simulink model "example_DHWconsumptionBasic"  (R2013b)
settings: Solver=ode45  StartTime=0.0  StopTime=24*3600  RelTol=1e-3
libraries: carnot x5
settings Model: Creator=drhf  LastModifiedBy=drhf
settings DataIOCC: SignalLoggingSaveFormat=ModelDataLogs
settings OptimizationCC: ExpressionDepthLimit=2147483647
settings DebuggingCC: FcnCallInpInsideContextMsg=UseLocalSettings  StateNameClashWarn=warning
settings GRTTargetCC: CombineOutputUpdateFcns=off  GRTInterface=on

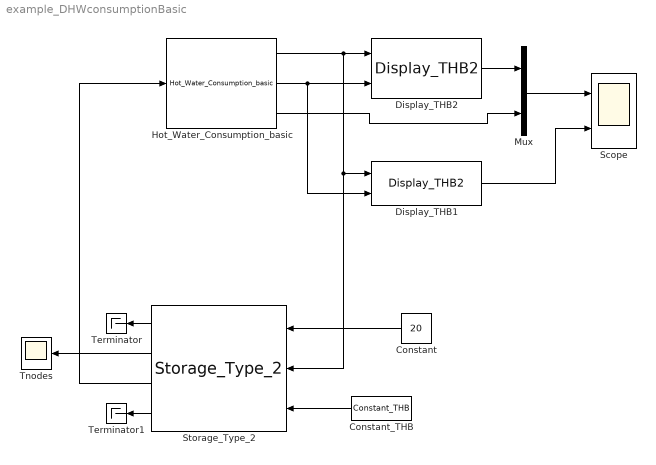
== system example_DHWconsumptionBasic ==
  Constant : Constant  Value=20
  Constant_THB : carnot/Source/Simple/Constant_THB  t=40  mdot=0*100/3600  p=1e5  mID=No Pressure Drop  fluid=Water  mix=0  mix2=0  mix3=0  dia=0.02  hgt=0
  Display_THB1 : carnot/Outputs/Display_THB2  t=off  m=on  p=off  id=off  mix=off  d=off
  Display_THB2 : carnot/Outputs/Display_THB2  t=on  m=off  p=off  id=off  mix=off  d=off
  Hot_Water_Consumption_basic : carnot/Load/Hot_Water_Tapping/Applications/Hot_Water_Consumption_basic  Thot=45  Tcold=10  period="24*3600   % one day"  time="[7 12 19]*3600  % tapping at 7:00, 12:00 and 19:00"  duration="[0.2 0.1 0.2]*3600  % in total 1/2 h tapping"  mdot="[1 1 1]*200/1800   % 200 kg in 1/2 h"
  Mux : Mux  Inputs=2
  Scope : Scope  NumInputPorts=2
      settings: YMin=5~0  YMax=55~0.12
  Storage_Type_2 : carnot/Storage/Thermal/Storage_Type_2  uloss=1  ubot=1  utop=1  cond=1  t0=60  volume=0.3  dia=0.5  pos=standing cylinder  nconnect=2  nodes=10  mpoints=10
  Terminator : Terminator
  Terminator1 : Terminator
  Tnodes : Scope
  wires:
  Hot_Water_Consumption_basic/2 -> Display_THB1/2, Display_THB2/2
  Display_THB2/1 -> Mux/1
  Hot_Water_Consumption_basic/3 -> Mux/2
  Mux/1 -> Scope/1
  Display_THB1/1 -> Scope/2
  Storage_Type_2/3 -> Hot_Water_Consumption_basic/1
  Hot_Water_Consumption_basic/1 -> Storage_Type_2/2, Display_THB1/1, Display_THB2/1
  Storage_Type_2/1 -> Terminator/1
  Storage_Type_2/4 -> Terminator1/1
  Constant_THB/1 -> Storage_Type_2/3
  Constant/1 -> Storage_Type_2/1
  Storage_Type_2/2 -> Tnodes/1
